simulink model "Three_Band_EQ_Model_r2018a"  (Simulink 9.1)
settings: Solver=FixedStepDiscrete  StartTime=0.0  StopTime=600  RelTol=1e-3  EnableMultiTasking=on
undefined symbols (not defined in the file): A1, A2, A3, B1, B2, B3, dfilt
libraries: dspobslib x4, dspvision x1
settings Model: Creator=mark  LastModifiedBy=Chris
settings DataIOCC: LimitDataPoints=on
settings OptimizationCC: ExpressionDepthLimit=2147483647
settings DebuggingCC: StateNameClashWarn=warning
settings GRTTargetCC: CombineOutputUpdateFcns=on  GRTInterface=off

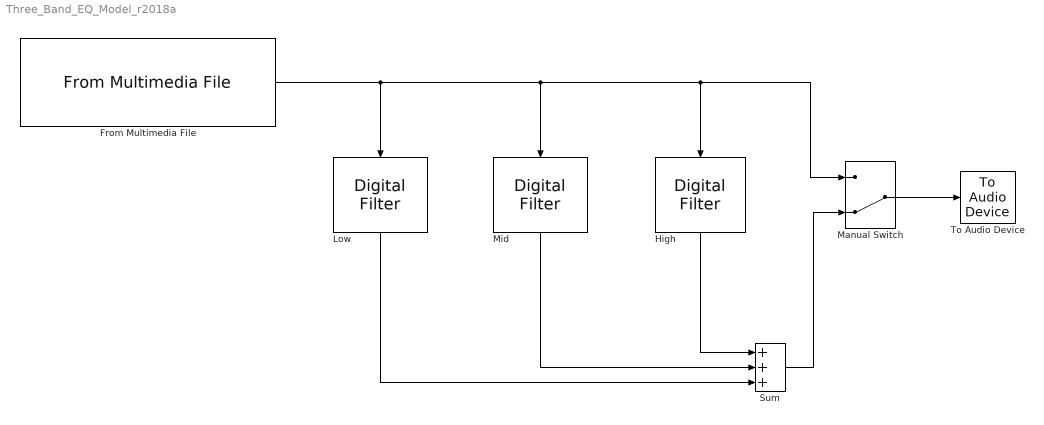
== system Three_Band_EQ_Model_r2018a ==
  From Multimedia File : dspvision/From Multimedia File  inputFilename=msmv2.wav  loop=on  numPlays=inf  outputStreams=Audio only  videoDataType=single  audioDataType=double  inheritSampleTime=on  userDefinedSampleTime=1/30  noAudioOutput=off  isIntensityVideo=off  fourcc=RGB  colorVideoFormat=Separate color signals  outputEOF=off  dataOrg=Column-major  audioFrameSize=1024  computeAudioFrameSize=off  outSamplingMode=Frame based
  "High  " : dspobslib/Digital Filter  TypePopup=IIR (poles & zeros)  IIRFiltStruct=Direct form II transposed  AllPoleFiltStruct=Direct form  FIRFiltStruct=Direct form  CoeffSource=Specify via dialog  NumCoeffs=[B3]  DenCoeffs=[A3]  BiQuadCoeffs=[1 0.3 0.4 1 0.1 0.2]  LatticeCoeffs=[0.2 0.4]  denIgnore=on  FiltPerSampPopup=One filter per frame  IC=0  ICnum=0  ICden=0  roundingMode=Floor  overflowMode=off  ScaleValues=1  scaleValueFracLength=14  stageInFracLength=15  stageOutFracLength=15  FilterSource=Specify via dialog  dfiltObjectName=dfilt.dffir([1 2 1])  InputProcessing=Columns as channels (frame based)
      settings: SourceProductBaseCode=DS
  "Low  " : dspobslib/Digital Filter  TypePopup=IIR (poles & zeros)  IIRFiltStruct=Direct form II transposed  AllPoleFiltStruct=Direct form  FIRFiltStruct=Direct form  CoeffSource=Specify via dialog  NumCoeffs=[B1 ]  DenCoeffs=[A1]  BiQuadCoeffs=[1 0.3 0.4 1 0.1 0.2]  LatticeCoeffs=[0.2 0.4]  denIgnore=on  FiltPerSampPopup=One filter per frame  IC=0  ICnum=0  ICden=0  roundingMode=Floor  overflowMode=off  ScaleValues=1  scaleValueFracLength=14  stageInFracLength=15  stageOutFracLength=15  FilterSource=Specify via dialog  dfiltObjectName=dfilt.dffir([1 2 1])  InputProcessing=Columns as channels (frame based)
      settings: SourceProductBaseCode=DS
  Manual Switch : ManualSwitch  CurrentSetting=0
  "Mid  " : dspobslib/Digital Filter  TypePopup=IIR (poles & zeros)  IIRFiltStruct=Direct form II transposed  AllPoleFiltStruct=Direct form  FIRFiltStruct=Direct form  CoeffSource=Specify via dialog  NumCoeffs=[B2]  DenCoeffs=[A2]  BiQuadCoeffs=[1 0.3 0.4 1 0.1 0.2]  LatticeCoeffs=[0.2 0.4]  denIgnore=on  FiltPerSampPopup=One filter per frame  IC=0  ICnum=0  ICden=0  roundingMode=Floor  overflowMode=off  ScaleValues=1  scaleValueFracLength=14  stageInFracLength=15  stageOutFracLength=15  FilterSource=Specify via dialog  dfiltObjectName=dfilt.dffir([1 2 1])  InputProcessing=Columns as channels (frame based)
      settings: SourceProductBaseCode=DS
  Sum : Sum  Inputs=+++
  To Audio Device : dspobslib/To Audio Device  deviceName=Built-in Output  inheritSampleRate=on  sampleRate=44100  deviceDatatype=Determine from input data type  autoBufferSize=on  bufferSize=4096  queueDuration=1.0  defaultOutputChannelMapping=on  outputChannelMapping=1:2  outputNumUnderrunSamples=off
      settings: SourceProductBaseCode=DS
  wires:
  Manual Switch/1 -> To Audio Device/1
  Sum/1 -> Manual Switch/2
  From Multimedia File/1 -> "Low  "/1, "Mid  "/1, Manual Switch/1, "High  "/1
  "Mid  "/1 -> Sum/2
  "Low  "/1 -> Sum/3
  "High  "/1 -> Sum/1
